simulink model "FactorialUsingWhileLoop"  (R2021a)
settings: Solver=FixedStepDiscrete  StartTime=0.0  StopTime=10  RelTol=1e-3
settings Model: Creator=OmarMedhat  LastModifiedBy=OmarMedhat
settings OptimizationCC: DefaultParameterBehavior=Inlined  EnhancedBackFolding=on  PassReuseOutputArgsAs=Individual arguments  ZeroExternalMemoryAtStartup=off  ZeroInternalMemoryAtStartup=off  OptimizeBlockOrder=speed  DifferentSizesBufferReuse=on  OptimizationCustomize=off  EfficientTunableParamExpr=on
settings DebuggingCC: ParameterTunabilityLossMsg=error
settings SFSimCC: MATLABDynamicMemAlloc=off
settings RTWCC: SystemTargetFile=ert.tlc  GenCodeOnly=on  TemplateMakefile=ert_default_tmf  GenerateReport=on  IncludeHyperlinkInReport=on  LaunchReport=on  GenerateTraceInfo=on
settings CodeAppCC: ForceParamTrailComments=on  IgnoreCustomStorageClasses=off  OperatorAnnotations=on  SimulinkDataObjDesc=on  SFDataObjDesc=on  InsertBlockDesc=on
settings ERTTargetCC: TargetLangStandard=C99 (ISO)  GenerateSampleERTMain=on  InlinedParameterPlacement=NonHierarchical  ERTCustomFileTemplate=example_file_process.tlc

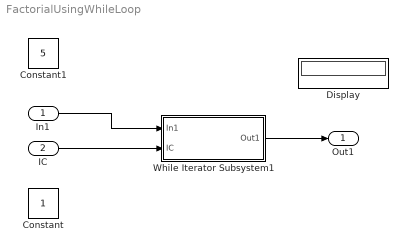
== system FactorialUsingWhileLoop ==
  In1 : Inport
  IC : Inport  Port=2
  Constant : Constant
  Constant1 : Constant  Value=5
  Display : Display
  While Iterator Subsystem1 : Subsystem  TreatAsAtomicUnit=on
  Out1 : Outport
  wires:
  In1/1 -> While Iterator Subsystem1/1(In1)
  IC/1 -> While Iterator Subsystem1/2(IC)
  While Iterator Subsystem1/1(Out1) -> Out1/1

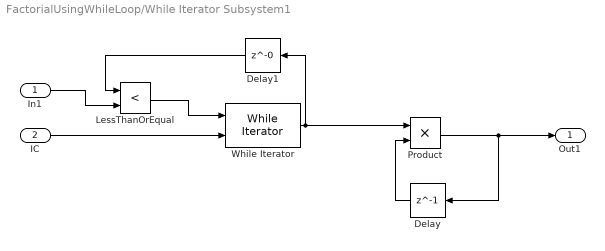
== system FactorialUsingWhileLoop/While Iterator Subsystem1 ==
  In1 : Inport
  IC : Inport  Port=2
  Delay : Delay  DelayLength=1  InitialCondition=1
  Delay1 : Delay  DelayLength=0  InitialCondition=0
  LessThanOrEqual : RelationalOperator  Operator=<  OutDataTypeStr=boolean  RndMeth=Simplest
  Product : Product  OutDataTypeStr=int32
  While Iterator : WhileIterator  MaxIters=-1  ShowIterationPort=on
  Out1 : Outport
  wires:
  IC/1 -> While Iterator/2
  While Iterator/1 -> Delay1/1, Product/1
  Product/1 -> Delay/1, Out1/1
  Delay/1 -> Product/2
  In1/1 -> LessThanOrEqual/2
  Delay1/1 -> LessThanOrEqual/1
  LessThanOrEqual/1 -> While Iterator/1
